simulink model "pasp_16i16c128s"  (Simulink 6.2)
settings: Solver=ode45  StartTime=0.0  StopTime=30000  RelTol=1e-3
undefined symbols (not defined in the file or in its folder): iBOB
libraries: xbsIndex_r3 x1501, casper_library x145, xps_library x90
(part 5 of 12)

== system pasp_16i16c128s/pasp/pfb_fir_real/pol1_in1_first_tap ==
  din : Inport  Port=1  LatchInput=off
  sync : Inport  Port=2  LatchInput=off
  Mult : xbsIndex_r3/Mult  precision=Full  arith_type="Signed  (2's comp)"  n_bits=8  bin_pt=2  quantization=Truncate  overflow=Wrap  latency=mult_latency  explicit_period=off  period=1  en=off  dbl_ovrd=off  show_param=on  mult_type=Parallel  oversample=2  use_embedded=on  pipeline=on  use_rpm=on  placement_style=Rectangular Shape  gen_core=off
      settings: xl_area=[0, 0, 0, 0, 0, 0, 0]
  Reinterpret : xbsIndex_r3/Reinterpret  force_arith_type=on  arith_type="Signed  (2's comp)"  force_bin_pt=on  bin_pt=CoeffBitWidth - 1  force_valid=on
  Reinterpret1 : xbsIndex_r3/Reinterpret  force_arith_type=on  arith_type=Unsigned  force_bin_pt=on  bin_pt=0  force_valid=on
  Reinterpret2 : xbsIndex_r3/Reinterpret  force_arith_type=on  arith_type="Signed  (2's comp)"  force_bin_pt=on  bin_pt=BitWidthIn - 1  force_valid=on
  Slice : xbsIndex_r3/Slice  mode=Lower Bit Location + Width  nbits=CoeffBitWidth  bit1=0  base1=MSB of Input  bit0=0  base0=LSB of Input  boolean_output=off  explicit_period=off  period=1  dbl_ovrd=off
  Slice1 : xbsIndex_r3/Slice  mode=Two Bit Locations  nbits=CoeffBitWidth * (TotalTaps - 1)  bit1=0  base1=MSB of Input  bit0=CoeffBitWidth  base0=LSB of Input  boolean_output=off  explicit_period=off  period=1  dbl_ovrd=off
  delay : Subsystem  BlockChoice=delay_bram
      link override delay_bram: DelayLen=2^(PFBSize-n_inputs)  bram_latency=bram_latency
      link override delay_bram/Constant2: equ=P=C
      settings: AttributesFormatString=%<BlockChoice>  TemplateBlock=casper_library/Delays/delay  MemberBlocks=delay_bram,delay_slr
  pfb_coeff_gen : Subsystem  AncestorBlock=casper_library/PFBs/pfb_coeff_gen  mask(pfb_coeff_gen){PFBSize=5, CoeffBitWidth=8, TotalTaps=2, CoeffDistMem=1, CoeffRound=0, WindowType=hamming, bram_latency=2, n_inputs=2, nput=0, fwidth=1}
      mask prompts: PFBSize "Size of PFB: (2^? pnts)"; CoeffBitWidth "Bitwidth of Coefficients:"; TotalTaps "Total Number of Taps:"; CoeffDistMem "Implement Coeff Gen in Distributed Memory"; CoeffRound "Round-off Coefficients"; WindowType "Windowing Function:"; bram_latency "BRAM Latency"; n_inputs "Number of Simultaneous Inputs: (2^?)"; nput "This is input number:"; fwidth "Bin Width (normal=1)"
      mask init:
      | pfb_coeff_gen_init(gcb, ...
      |     'PFBSize', PFBSize, ...
      |     'CoeffBitWidth', CoeffBitWidth, ...
      |     'CoeffRound', CoeffRound, ...
      |     'TotalTaps', TotalTaps, ...
      |     'CoeffDistMem', CoeffDistMem, ...
      |     'WindowType', WindowType, ...
      |     'bram_latency', bram_latency, ...
      |     'n_inputs', n_inputs, ...
      |     'nput', nput, ...
      |     'fwidth', fwidth);
      settings: AttributesFormatString=PFBSize=5, n_inputs=2, taps=2
  sync_delay : casper_library/Delays/sync_delay  DelayLen=2^(PFBSize-n_inputs)
      link override Constant: equ=P=C
      link override Constant1: equ=P=C
      link override Constant2: equ=P=C
      link override Constant3: equ=P=C
  dout : Outport
  sync_out : Outport  Port=2
  coeff_out : Outport  Port=3
  taps_out : Outport  Port=4
  wires:
  Reinterpret2/1 -> Mult/1
  Reinterpret1/1 -> taps_out/1
  Reinterpret/1 -> Mult/2
  Slice/1 -> Reinterpret/1
  Slice1/1 -> coeff_out/1
  sync_delay/1 -> sync_out/1
  delay/1(Out1) -> dout/1
  pfb_coeff_gen/1(dout) -> delay/1(In1), Reinterpret2/1
  pfb_coeff_gen/2(sync_out) -> sync_delay/1
  pfb_coeff_gen/3(coeff) -> Slice/1, Slice1/1
  Mult/1 -> Reinterpret1/1
  din/1 -> pfb_coeff_gen/1(din)
  sync/1 -> pfb_coeff_gen/2(sync)

== system pasp_16i16c128s/pasp/pfb_fir_real/pol1_in1_last_tap ==
  din : Inport  Port=1  LatchInput=off
  sync : Inport  Port=2  LatchInput=off
  coeff : Inport  Port=3  LatchInput=off
  taps : Inport  Port=4  LatchInput=off
  Concat : xbsIndex_r3/Concat  num_inputs=2  explicit_period=off  period=1  dbl_ovrd=off
  Delay : xbsIndex_r3/Delay  latency=mult_latency  reg_retiming=off  explicit_period=off  period=1  en=off  accept_only_valid=off  init_zero=on  dbl_ovrd=off  show_param=off
      settings: xl_area=[0, 0, 0, 0, 0, 0, 0]
  Mult : xbsIndex_r3/Mult  precision=Full  arith_type="Signed  (2's comp)"  n_bits=8  bin_pt=2  quantization=Truncate  overflow=Wrap  latency=mult_latency  explicit_period=off  period=1  en=off  dbl_ovrd=off  show_param=on  mult_type=Parallel  oversample=2  use_embedded=on  pipeline=on  use_rpm=on  placement_style=Rectangular Shape  gen_core=off
      settings: xl_area=[0, 0, 0, 0, 0, 0, 0]
  Reinterpret : xbsIndex_r3/Reinterpret  force_arith_type=on  arith_type="Signed  (2's comp)"  force_bin_pt=on  bin_pt=CoeffBitWidth - 1  force_valid=on
  Reinterpret1 : xbsIndex_r3/Reinterpret  force_arith_type=on  arith_type="Signed  (2's comp)"  force_bin_pt=on  bin_pt=BitWidthIn - 1  force_valid=on
  Reinterpret2 : xbsIndex_r3/Reinterpret  force_arith_type=on  arith_type=Unsigned  force_bin_pt=on  bin_pt=0  force_valid=on
  pfb_real_add_tree : Subsystem  mask(pfb_real_add_tree){TotalTaps=2, BitWidthIn=8, BitWidthOut=18, CoeffBitWidth=8, add_latency=1, quantization=Truncate}
      mask prompts: TotalTaps "Total Number of Taps:"; BitWidthIn "Input Bitwidth:"; BitWidthOut "Output Bitwidth:"; CoeffBitWidth "Coeff Bitwidth:"; add_latency "Add Latency"; quantization "Quantization Behavior"
      mask init:
      | pfb_real_add_tree_init(gcb, ...
      |     'TotalTaps', TotalTaps, ...
      |     'BitWidthIn', BitWidthIn, ...
      |     'BitWidthOut', BitWidthOut, ...
      |     'CoeffBitWidth', CoeffBitWidth, ...
      |     'add_latency', add_latency, ...
      |     'quantization', quantization);
      settings: AttributesFormatString=taps=2, add_latency=1
  dout : Outport
  sync_out : Outport  Port=2
  wires:
  Delay/1 -> pfb_real_add_tree/2(sync)
  pfb_real_add_tree/2(sync_out) -> sync_out/1
  din/1 -> Reinterpret1/1
  sync/1 -> Delay/1
  taps/1 -> Concat/2
  Concat/1 -> pfb_real_add_tree/1(din)
  coeff/1 -> Reinterpret/1
  Reinterpret/1 -> Mult/2
  Mult/1 -> Reinterpret2/1
  Reinterpret1/1 -> Mult/1
  Reinterpret2/1 -> Concat/1
  pfb_real_add_tree/1(dout) -> dout/1

== system pasp_16i16c128s/pasp/pfb_fir_real/pol1_in2_first_tap ==
  din : Inport  Port=1  LatchInput=off
  sync : Inport  Port=2  LatchInput=off
  Mult : xbsIndex_r3/Mult  precision=Full  arith_type="Signed  (2's comp)"  n_bits=8  bin_pt=2  quantization=Truncate  overflow=Wrap  latency=mult_latency  explicit_period=off  period=1  en=off  dbl_ovrd=off  show_param=on  mult_type=Parallel  oversample=2  use_embedded=on  pipeline=on  use_rpm=on  placement_style=Rectangular Shape  gen_core=off
      settings: xl_area=[0, 0, 0, 0, 0, 0, 0]
  Reinterpret : xbsIndex_r3/Reinterpret  force_arith_type=on  arith_type="Signed  (2's comp)"  force_bin_pt=on  bin_pt=CoeffBitWidth - 1  force_valid=on
  Reinterpret1 : xbsIndex_r3/Reinterpret  force_arith_type=on  arith_type=Unsigned  force_bin_pt=on  bin_pt=0  force_valid=on
  Reinterpret2 : xbsIndex_r3/Reinterpret  force_arith_type=on  arith_type="Signed  (2's comp)"  force_bin_pt=on  bin_pt=BitWidthIn - 1  force_valid=on
  Slice : xbsIndex_r3/Slice  mode=Lower Bit Location + Width  nbits=CoeffBitWidth  bit1=0  base1=MSB of Input  bit0=0  base0=LSB of Input  boolean_output=off  explicit_period=off  period=1  dbl_ovrd=off
  Slice1 : xbsIndex_r3/Slice  mode=Two Bit Locations  nbits=CoeffBitWidth * (TotalTaps - 1)  bit1=0  base1=MSB of Input  bit0=CoeffBitWidth  base0=LSB of Input  boolean_output=off  explicit_period=off  period=1  dbl_ovrd=off
  delay : Subsystem  BlockChoice=delay_bram
      link override delay_bram: DelayLen=2^(PFBSize-n_inputs)  bram_latency=bram_latency
      link override delay_bram/Constant2: equ=P=C
      settings: AttributesFormatString=%<BlockChoice>  TemplateBlock=casper_library/Delays/delay  MemberBlocks=delay_bram,delay_slr
  pfb_coeff_gen : Subsystem  AncestorBlock=casper_library/PFBs/pfb_coeff_gen  mask(pfb_coeff_gen){PFBSize=5, CoeffBitWidth=8, TotalTaps=2, CoeffDistMem=1, CoeffRound=0, WindowType=hamming, bram_latency=2, n_inputs=2, nput=1, fwidth=1}
      mask prompts: PFBSize "Size of PFB: (2^? pnts)"; CoeffBitWidth "Bitwidth of Coefficients:"; TotalTaps "Total Number of Taps:"; CoeffDistMem "Implement Coeff Gen in Distributed Memory"; CoeffRound "Round-off Coefficients"; WindowType "Windowing Function:"; bram_latency "BRAM Latency"; n_inputs "Number of Simultaneous Inputs: (2^?)"; nput "This is input number:"; fwidth "Bin Width (normal=1)"
      mask init: same as pasp_16i16c128s/pasp/pfb_fir_real/pol1_in1_first_tap/pfb_coeff_gen
      settings: AttributesFormatString=PFBSize=5, n_inputs=2, taps=2
  sync_delay : casper_library/Delays/sync_delay  DelayLen=2^(PFBSize-n_inputs)
      link override Constant: equ=P=C
      link override Constant1: equ=P=C
      link override Constant2: equ=P=C
      link override Constant3: equ=P=C
  dout : Outport
  sync_out : Outport  Port=2
  coeff_out : Outport  Port=3
  taps_out : Outport  Port=4
  wires:
  Reinterpret2/1 -> Mult/1
  Reinterpret1/1 -> taps_out/1
  Reinterpret/1 -> Mult/2
  Slice/1 -> Reinterpret/1
  Slice1/1 -> coeff_out/1
  sync_delay/1 -> sync_out/1
  delay/1(Out1) -> dout/1
  pfb_coeff_gen/1(dout) -> delay/1(In1), Reinterpret2/1
  pfb_coeff_gen/2(sync_out) -> sync_delay/1
  pfb_coeff_gen/3(coeff) -> Slice/1, Slice1/1
  Mult/1 -> Reinterpret1/1
  din/1 -> pfb_coeff_gen/1(din)
  sync/1 -> pfb_coeff_gen/2(sync)

== system pasp_16i16c128s/pasp/pfb_fir_real/pol1_in2_last_tap ==
  din : Inport  Port=1  LatchInput=off
  sync : Inport  Port=2  LatchInput=off
  coeff : Inport  Port=3  LatchInput=off
  taps : Inport  Port=4  LatchInput=off
  Concat : xbsIndex_r3/Concat  num_inputs=2  explicit_period=off  period=1  dbl_ovrd=off
  Delay : xbsIndex_r3/Delay  latency=mult_latency  reg_retiming=off  explicit_period=off  period=1  en=off  accept_only_valid=off  init_zero=on  dbl_ovrd=off  show_param=off
      settings: xl_area=[0, 0, 0, 0, 0, 0, 0]
  Mult : xbsIndex_r3/Mult  precision=Full  arith_type="Signed  (2's comp)"  n_bits=8  bin_pt=2  quantization=Truncate  overflow=Wrap  latency=mult_latency  explicit_period=off  period=1  en=off  dbl_ovrd=off  show_param=on  mult_type=Parallel  oversample=2  use_embedded=on  pipeline=on  use_rpm=on  placement_style=Rectangular Shape  gen_core=off
      settings: xl_area=[0, 0, 0, 0, 0, 0, 0]
  Reinterpret : xbsIndex_r3/Reinterpret  force_arith_type=on  arith_type="Signed  (2's comp)"  force_bin_pt=on  bin_pt=CoeffBitWidth - 1  force_valid=on
  Reinterpret1 : xbsIndex_r3/Reinterpret  force_arith_type=on  arith_type="Signed  (2's comp)"  force_bin_pt=on  bin_pt=BitWidthIn - 1  force_valid=on
  Reinterpret2 : xbsIndex_r3/Reinterpret  force_arith_type=on  arith_type=Unsigned  force_bin_pt=on  bin_pt=0  force_valid=on
  pfb_real_add_tree : Subsystem  mask(pfb_real_add_tree){TotalTaps=2, BitWidthIn=8, BitWidthOut=18, CoeffBitWidth=8, add_latency=1, quantization=Truncate}
      mask prompts: TotalTaps "Total Number of Taps:"; BitWidthIn "Input Bitwidth:"; BitWidthOut "Output Bitwidth:"; CoeffBitWidth "Coeff Bitwidth:"; add_latency "Add Latency"; quantization "Quantization Behavior"
      mask init: same as pasp_16i16c128s/pasp/pfb_fir_real/pol1_in1_last_tap/pfb_real_add_tree
      settings: AttributesFormatString=taps=2, add_latency=1
  dout : Outport
  sync_out : Outport  Port=2
  wires:
  Delay/1 -> pfb_real_add_tree/2(sync)
  pfb_real_add_tree/2(sync_out) -> sync_out/1
  din/1 -> Reinterpret1/1
  sync/1 -> Delay/1
  taps/1 -> Concat/2
  Concat/1 -> pfb_real_add_tree/1(din)
  coeff/1 -> Reinterpret/1
  Reinterpret/1 -> Mult/2
  Mult/1 -> Reinterpret2/1
  Reinterpret1/1 -> Mult/1
  Reinterpret2/1 -> Concat/1
  pfb_real_add_tree/1(dout) -> dout/1

== system pasp_16i16c128s/pasp/pfb_fir_real/pol1_in3_first_tap ==
  din : Inport  Port=1  LatchInput=off
  sync : Inport  Port=2  LatchInput=off
  Mult : xbsIndex_r3/Mult  precision=Full  arith_type="Signed  (2's comp)"  n_bits=8  bin_pt=2  quantization=Truncate  overflow=Wrap  latency=mult_latency  explicit_period=off  period=1  en=off  dbl_ovrd=off  show_param=on  mult_type=Parallel  oversample=2  use_embedded=on  pipeline=on  use_rpm=on  placement_style=Rectangular Shape  gen_core=off
      settings: xl_area=[0, 0, 0, 0, 0, 0, 0]
  Reinterpret : xbsIndex_r3/Reinterpret  force_arith_type=on  arith_type="Signed  (2's comp)"  force_bin_pt=on  bin_pt=CoeffBitWidth - 1  force_valid=on
  Reinterpret1 : xbsIndex_r3/Reinterpret  force_arith_type=on  arith_type=Unsigned  force_bin_pt=on  bin_pt=0  force_valid=on
  Reinterpret2 : xbsIndex_r3/Reinterpret  force_arith_type=on  arith_type="Signed  (2's comp)"  force_bin_pt=on  bin_pt=BitWidthIn - 1  force_valid=on
  Slice : xbsIndex_r3/Slice  mode=Lower Bit Location + Width  nbits=CoeffBitWidth  bit1=0  base1=MSB of Input  bit0=0  base0=LSB of Input  boolean_output=off  explicit_period=off  period=1  dbl_ovrd=off
  Slice1 : xbsIndex_r3/Slice  mode=Two Bit Locations  nbits=CoeffBitWidth * (TotalTaps - 1)  bit1=0  base1=MSB of Input  bit0=CoeffBitWidth  base0=LSB of Input  boolean_output=off  explicit_period=off  period=1  dbl_ovrd=off
  delay : Subsystem  BlockChoice=delay_bram
      link override delay_bram: DelayLen=2^(PFBSize-n_inputs)  bram_latency=bram_latency
      link override delay_bram/Constant2: equ=P=C
      settings: AttributesFormatString=%<BlockChoice>  TemplateBlock=casper_library/Delays/delay  MemberBlocks=delay_bram,delay_slr
  pfb_coeff_gen : Subsystem  AncestorBlock=casper_library/PFBs/pfb_coeff_gen  mask(pfb_coeff_gen){PFBSize=5, CoeffBitWidth=8, TotalTaps=2, CoeffDistMem=1, CoeffRound=0, WindowType=hamming, bram_latency=2, n_inputs=2, nput=2, fwidth=1}
      mask prompts: PFBSize "Size of PFB: (2^? pnts)"; CoeffBitWidth "Bitwidth of Coefficients:"; TotalTaps "Total Number of Taps:"; CoeffDistMem "Implement Coeff Gen in Distributed Memory"; CoeffRound "Round-off Coefficients"; WindowType "Windowing Function:"; bram_latency "BRAM Latency"; n_inputs "Number of Simultaneous Inputs: (2^?)"; nput "This is input number:"; fwidth "Bin Width (normal=1)"
      mask init: same as pasp_16i16c128s/pasp/pfb_fir_real/pol1_in1_first_tap/pfb_coeff_gen
      settings: AttributesFormatString=PFBSize=5, n_inputs=2, taps=2
  sync_delay : casper_library/Delays/sync_delay  DelayLen=2^(PFBSize-n_inputs)
      link override Constant: equ=P=C
      link override Constant1: equ=P=C
      link override Constant2: equ=P=C
      link override Constant3: equ=P=C
  dout : Outport
  sync_out : Outport  Port=2
  coeff_out : Outport  Port=3
  taps_out : Outport  Port=4
  wires:
  Reinterpret2/1 -> Mult/1
  Reinterpret1/1 -> taps_out/1
  Reinterpret/1 -> Mult/2
  Slice/1 -> Reinterpret/1
  Slice1/1 -> coeff_out/1
  sync_delay/1 -> sync_out/1
  delay/1(Out1) -> dout/1
  pfb_coeff_gen/1(dout) -> delay/1(In1), Reinterpret2/1
  pfb_coeff_gen/2(sync_out) -> sync_delay/1
  pfb_coeff_gen/3(coeff) -> Slice/1, Slice1/1
  Mult/1 -> Reinterpret1/1
  din/1 -> pfb_coeff_gen/1(din)
  sync/1 -> pfb_coeff_gen/2(sync)

== system pasp_16i16c128s/pasp/pfb_fir_real/pol1_in3_last_tap ==
  din : Inport  Port=1  LatchInput=off
  sync : Inport  Port=2  LatchInput=off
  coeff : Inport  Port=3  LatchInput=off
  taps : Inport  Port=4  LatchInput=off
  Concat : xbsIndex_r3/Concat  num_inputs=2  explicit_period=off  period=1  dbl_ovrd=off
  Delay : xbsIndex_r3/Delay  latency=mult_latency  reg_retiming=off  explicit_period=off  period=1  en=off  accept_only_valid=off  init_zero=on  dbl_ovrd=off  show_param=off
      settings: xl_area=[0, 0, 0, 0, 0, 0, 0]
  Mult : xbsIndex_r3/Mult  precision=Full  arith_type="Signed  (2's comp)"  n_bits=8  bin_pt=2  quantization=Truncate  overflow=Wrap  latency=mult_latency  explicit_period=off  period=1  en=off  dbl_ovrd=off  show_param=on  mult_type=Parallel  oversample=2  use_embedded=on  pipeline=on  use_rpm=on  placement_style=Rectangular Shape  gen_core=off
      settings: xl_area=[0, 0, 0, 0, 0, 0, 0]
  Reinterpret : xbsIndex_r3/Reinterpret  force_arith_type=on  arith_type="Signed  (2's comp)"  force_bin_pt=on  bin_pt=CoeffBitWidth - 1  force_valid=on
  Reinterpret1 : xbsIndex_r3/Reinterpret  force_arith_type=on  arith_type="Signed  (2's comp)"  force_bin_pt=on  bin_pt=BitWidthIn - 1  force_valid=on
  Reinterpret2 : xbsIndex_r3/Reinterpret  force_arith_type=on  arith_type=Unsigned  force_bin_pt=on  bin_pt=0  force_valid=on
  pfb_real_add_tree : Subsystem  mask(pfb_real_add_tree){TotalTaps=2, BitWidthIn=8, BitWidthOut=18, CoeffBitWidth=8, add_latency=1, quantization=Truncate}
      mask prompts: TotalTaps "Total Number of Taps:"; BitWidthIn "Input Bitwidth:"; BitWidthOut "Output Bitwidth:"; CoeffBitWidth "Coeff Bitwidth:"; add_latency "Add Latency"; quantization "Quantization Behavior"
      mask init: same as pasp_16i16c128s/pasp/pfb_fir_real/pol1_in1_last_tap/pfb_real_add_tree
      settings: AttributesFormatString=taps=2, add_latency=1
  dout : Outport
  sync_out : Outport  Port=2
  wires:
  Delay/1 -> pfb_real_add_tree/2(sync)
  pfb_real_add_tree/2(sync_out) -> sync_out/1
  din/1 -> Reinterpret1/1
  sync/1 -> Delay/1
  taps/1 -> Concat/2
  Concat/1 -> pfb_real_add_tree/1(din)
  coeff/1 -> Reinterpret/1
  Reinterpret/1 -> Mult/2
  Mult/1 -> Reinterpret2/1
  Reinterpret1/1 -> Mult/1
  Reinterpret2/1 -> Concat/1
  pfb_real_add_tree/1(dout) -> dout/1

== system pasp_16i16c128s/pasp/pfb_fir_real/pol1_in4_first_tap ==
  din : Inport  Port=1  LatchInput=off
  sync : Inport  Port=2  LatchInput=off
  Mult : xbsIndex_r3/Mult  precision=Full  arith_type="Signed  (2's comp)"  n_bits=8  bin_pt=2  quantization=Truncate  overflow=Wrap  latency=mult_latency  explicit_period=off  period=1  en=off  dbl_ovrd=off  show_param=on  mult_type=Parallel  oversample=2  use_embedded=on  pipeline=on  use_rpm=on  placement_style=Rectangular Shape  gen_core=off
      settings: xl_area=[0, 0, 0, 0, 0, 0, 0]
  Reinterpret : xbsIndex_r3/Reinterpret  force_arith_type=on  arith_type="Signed  (2's comp)"  force_bin_pt=on  bin_pt=CoeffBitWidth - 1  force_valid=on
  Reinterpret1 : xbsIndex_r3/Reinterpret  force_arith_type=on  arith_type=Unsigned  force_bin_pt=on  bin_pt=0  force_valid=on
  Reinterpret2 : xbsIndex_r3/Reinterpret  force_arith_type=on  arith_type="Signed  (2's comp)"  force_bin_pt=on  bin_pt=BitWidthIn - 1  force_valid=on
  Slice : xbsIndex_r3/Slice  mode=Lower Bit Location + Width  nbits=CoeffBitWidth  bit1=0  base1=MSB of Input  bit0=0  base0=LSB of Input  boolean_output=off  explicit_period=off  period=1  dbl_ovrd=off
  Slice1 : xbsIndex_r3/Slice  mode=Two Bit Locations  nbits=CoeffBitWidth * (TotalTaps - 1)  bit1=0  base1=MSB of Input  bit0=CoeffBitWidth  base0=LSB of Input  boolean_output=off  explicit_period=off  period=1  dbl_ovrd=off
  delay : Subsystem  BlockChoice=delay_bram
      link override delay_bram: DelayLen=2^(PFBSize-n_inputs)  bram_latency=bram_latency
      link override delay_bram/Constant2: equ=P=C
      settings: AttributesFormatString=%<BlockChoice>  TemplateBlock=casper_library/Delays/delay  MemberBlocks=delay_bram,delay_slr
  pfb_coeff_gen : Subsystem  AncestorBlock=casper_library/PFBs/pfb_coeff_gen  mask(pfb_coeff_gen){PFBSize=5, CoeffBitWidth=8, TotalTaps=2, CoeffDistMem=1, CoeffRound=0, WindowType=hamming, bram_latency=2, n_inputs=2, nput=3, fwidth=1}
      mask prompts: PFBSize "Size of PFB: (2^? pnts)"; CoeffBitWidth "Bitwidth of Coefficients:"; TotalTaps "Total Number of Taps:"; CoeffDistMem "Implement Coeff Gen in Distributed Memory"; CoeffRound "Round-off Coefficients"; WindowType "Windowing Function:"; bram_latency "BRAM Latency"; n_inputs "Number of Simultaneous Inputs: (2^?)"; nput "This is input number:"; fwidth "Bin Width (normal=1)"
      mask init: same as pasp_16i16c128s/pasp/pfb_fir_real/pol1_in1_first_tap/pfb_coeff_gen
      settings: AttributesFormatString=PFBSize=5, n_inputs=2, taps=2
  sync_delay : casper_library/Delays/sync_delay  DelayLen=2^(PFBSize-n_inputs)
      link override Constant: equ=P=C
      link override Constant1: equ=P=C
      link override Constant2: equ=P=C
      link override Constant3: equ=P=C
  dout : Outport
  sync_out : Outport  Port=2
  coeff_out : Outport  Port=3
  taps_out : Outport  Port=4
  wires:
  Reinterpret2/1 -> Mult/1
  Reinterpret1/1 -> taps_out/1
  Reinterpret/1 -> Mult/2
  Slice/1 -> Reinterpret/1
  Slice1/1 -> coeff_out/1
  sync_delay/1 -> sync_out/1
  delay/1(Out1) -> dout/1
  pfb_coeff_gen/1(dout) -> delay/1(In1), Reinterpret2/1
  pfb_coeff_gen/2(sync_out) -> sync_delay/1
  pfb_coeff_gen/3(coeff) -> Slice/1, Slice1/1
  Mult/1 -> Reinterpret1/1
  din/1 -> pfb_coeff_gen/1(din)
  sync/1 -> pfb_coeff_gen/2(sync)

== system pasp_16i16c128s/pasp/pfb_fir_real/pol1_in4_last_tap ==
  din : Inport  Port=1  LatchInput=off
  sync : Inport  Port=2  LatchInput=off
  coeff : Inport  Port=3  LatchInput=off
  taps : Inport  Port=4  LatchInput=off
  Concat : xbsIndex_r3/Concat  num_inputs=2  explicit_period=off  period=1  dbl_ovrd=off
  Delay : xbsIndex_r3/Delay  latency=mult_latency  reg_retiming=off  explicit_period=off  period=1  en=off  accept_only_valid=off  init_zero=on  dbl_ovrd=off  show_param=off
      settings: xl_area=[0, 0, 0, 0, 0, 0, 0]
  Mult : xbsIndex_r3/Mult  precision=Full  arith_type="Signed  (2's comp)"  n_bits=8  bin_pt=2  quantization=Truncate  overflow=Wrap  latency=mult_latency  explicit_period=off  period=1  en=off  dbl_ovrd=off  show_param=on  mult_type=Parallel  oversample=2  use_embedded=on  pipeline=on  use_rpm=on  placement_style=Rectangular Shape  gen_core=off
      settings: xl_area=[0, 0, 0, 0, 0, 0, 0]
  Reinterpret : xbsIndex_r3/Reinterpret  force_arith_type=on  arith_type="Signed  (2's comp)"  force_bin_pt=on  bin_pt=CoeffBitWidth - 1  force_valid=on
  Reinterpret1 : xbsIndex_r3/Reinterpret  force_arith_type=on  arith_type="Signed  (2's comp)"  force_bin_pt=on  bin_pt=BitWidthIn - 1  force_valid=on
  Reinterpret2 : xbsIndex_r3/Reinterpret  force_arith_type=on  arith_type=Unsigned  force_bin_pt=on  bin_pt=0  force_valid=on
  pfb_real_add_tree : Subsystem  mask(pfb_real_add_tree){TotalTaps=2, BitWidthIn=8, BitWidthOut=18, CoeffBitWidth=8, add_latency=1, quantization=Truncate}
      mask prompts: TotalTaps "Total Number of Taps:"; BitWidthIn "Input Bitwidth:"; BitWidthOut "Output Bitwidth:"; CoeffBitWidth "Coeff Bitwidth:"; add_latency "Add Latency"; quantization "Quantization Behavior"
      mask init: same as pasp_16i16c128s/pasp/pfb_fir_real/pol1_in1_last_tap/pfb_real_add_tree
      settings: AttributesFormatString=taps=2, add_latency=1
  dout : Outport
  sync_out : Outport  Port=2
  wires:
  Delay/1 -> pfb_real_add_tree/2(sync)
  pfb_real_add_tree/2(sync_out) -> sync_out/1
  din/1 -> Reinterpret1/1
  sync/1 -> Delay/1
  taps/1 -> Concat/2
  Concat/1 -> pfb_real_add_tree/1(din)
  coeff/1 -> Reinterpret/1
  Reinterpret/1 -> Mult/2
  Mult/1 -> Reinterpret2/1
  Reinterpret1/1 -> Mult/1
  Reinterpret2/1 -> Concat/1
  pfb_real_add_tree/1(dout) -> dout/1

== system pasp_16i16c128s/pasp/pfb_fir_real1/pol1_in1_first_tap ==
  din : Inport  Port=1  LatchInput=off
  sync : Inport  Port=2  LatchInput=off
  Mult : xbsIndex_r3/Mult  precision=Full  arith_type="Signed  (2's comp)"  n_bits=8  bin_pt=2  quantization=Truncate  overflow=Wrap  latency=mult_latency  explicit_period=off  period=1  en=off  dbl_ovrd=off  show_param=on  mult_type=Parallel  oversample=2  use_embedded=on  pipeline=on  use_rpm=on  placement_style=Rectangular Shape  gen_core=off
      settings: xl_area=[0, 0, 0, 0, 0, 0, 0]
  Reinterpret : xbsIndex_r3/Reinterpret  force_arith_type=on  arith_type="Signed  (2's comp)"  force_bin_pt=on  bin_pt=CoeffBitWidth - 1  force_valid=on
  Reinterpret1 : xbsIndex_r3/Reinterpret  force_arith_type=on  arith_type=Unsigned  force_bin_pt=on  bin_pt=0  force_valid=on
  Reinterpret2 : xbsIndex_r3/Reinterpret  force_arith_type=on  arith_type="Signed  (2's comp)"  force_bin_pt=on  bin_pt=BitWidthIn - 1  force_valid=on
  Slice : xbsIndex_r3/Slice  mode=Lower Bit Location + Width  nbits=CoeffBitWidth  bit1=0  base1=MSB of Input  bit0=0  base0=LSB of Input  boolean_output=off  explicit_period=off  period=1  dbl_ovrd=off
  Slice1 : xbsIndex_r3/Slice  mode=Two Bit Locations  nbits=CoeffBitWidth * (TotalTaps - 1)  bit1=0  base1=MSB of Input  bit0=CoeffBitWidth  base0=LSB of Input  boolean_output=off  explicit_period=off  period=1  dbl_ovrd=off
  delay : Subsystem  BlockChoice=delay_bram
      link override delay_bram: DelayLen=2^(PFBSize-n_inputs)  bram_latency=bram_latency
      link override delay_bram/Constant2: equ=P=C
      settings: AttributesFormatString=%<BlockChoice>  TemplateBlock=casper_library/Delays/delay  MemberBlocks=delay_bram,delay_slr
  pfb_coeff_gen : Subsystem  AncestorBlock=casper_library/PFBs/pfb_coeff_gen  mask(pfb_coeff_gen){PFBSize=5, CoeffBitWidth=8, TotalTaps=2, CoeffDistMem=1, CoeffRound=0, WindowType=hamming, bram_latency=2, n_inputs=2, nput=0, fwidth=1}
      mask prompts: PFBSize "Size of PFB: (2^? pnts)"; CoeffBitWidth "Bitwidth of Coefficients:"; TotalTaps "Total Number of Taps:"; CoeffDistMem "Implement Coeff Gen in Distributed Memory"; CoeffRound "Round-off Coefficients"; WindowType "Windowing Function:"; bram_latency "BRAM Latency"; n_inputs "Number of Simultaneous Inputs: (2^?)"; nput "This is input number:"; fwidth "Bin Width (normal=1)"
      mask init: same as pasp_16i16c128s/pasp/pfb_fir_real/pol1_in1_first_tap/pfb_coeff_gen
      settings: AttributesFormatString=PFBSize=5, n_inputs=2, taps=2
  sync_delay : casper_library/Delays/sync_delay  DelayLen=2^(PFBSize-n_inputs)
      link override Constant: equ=P=C
      link override Constant1: equ=P=C
      link override Constant2: equ=P=C
      link override Constant3: equ=P=C
  dout : Outport
  sync_out : Outport  Port=2
  coeff_out : Outport  Port=3
  taps_out : Outport  Port=4
  wires:
  Reinterpret2/1 -> Mult/1
  Reinterpret1/1 -> taps_out/1
  Reinterpret/1 -> Mult/2
  Slice/1 -> Reinterpret/1
  Slice1/1 -> coeff_out/1
  sync_delay/1 -> sync_out/1
  delay/1(Out1) -> dout/1
  pfb_coeff_gen/1(dout) -> delay/1(In1), Reinterpret2/1
  pfb_coeff_gen/2(sync_out) -> sync_delay/1
  pfb_coeff_gen/3(coeff) -> Slice/1, Slice1/1
  Mult/1 -> Reinterpret1/1
  din/1 -> pfb_coeff_gen/1(din)
  sync/1 -> pfb_coeff_gen/2(sync)

== system pasp_16i16c128s/pasp/pfb_fir_real1/pol1_in1_last_tap ==
  din : Inport  Port=1  LatchInput=off
  sync : Inport  Port=2  LatchInput=off
  coeff : Inport  Port=3  LatchInput=off
  taps : Inport  Port=4  LatchInput=off
  Concat : xbsIndex_r3/Concat  num_inputs=2  explicit_period=off  period=1  dbl_ovrd=off
  Delay : xbsIndex_r3/Delay  latency=mult_latency  reg_retiming=off  explicit_period=off  period=1  en=off  accept_only_valid=off  init_zero=on  dbl_ovrd=off  show_param=off
      settings: xl_area=[0, 0, 0, 0, 0, 0, 0]
  Mult : xbsIndex_r3/Mult  precision=Full  arith_type="Signed  (2's comp)"  n_bits=8  bin_pt=2  quantization=Truncate  overflow=Wrap  latency=mult_latency  explicit_period=off  period=1  en=off  dbl_ovrd=off  show_param=on  mult_type=Parallel  oversample=2  use_embedded=on  pipeline=on  use_rpm=on  placement_style=Rectangular Shape  gen_core=off
      settings: xl_area=[0, 0, 0, 0, 0, 0, 0]
  Reinterpret : xbsIndex_r3/Reinterpret  force_arith_type=on  arith_type="Signed  (2's comp)"  force_bin_pt=on  bin_pt=CoeffBitWidth - 1  force_valid=on
  Reinterpret1 : xbsIndex_r3/Reinterpret  force_arith_type=on  arith_type="Signed  (2's comp)"  force_bin_pt=on  bin_pt=BitWidthIn - 1  force_valid=on
  Reinterpret2 : xbsIndex_r3/Reinterpret  force_arith_type=on  arith_type=Unsigned  force_bin_pt=on  bin_pt=0  force_valid=on
  pfb_real_add_tree : Subsystem  mask(pfb_real_add_tree){TotalTaps=2, BitWidthIn=8, BitWidthOut=18, CoeffBitWidth=8, add_latency=1, quantization=Truncate}
      mask prompts: TotalTaps "Total Number of Taps:"; BitWidthIn "Input Bitwidth:"; BitWidthOut "Output Bitwidth:"; CoeffBitWidth "Coeff Bitwidth:"; add_latency "Add Latency"; quantization "Quantization Behavior"
      mask init: same as pasp_16i16c128s/pasp/pfb_fir_real/pol1_in1_last_tap/pfb_real_add_tree
      settings: AttributesFormatString=taps=2, add_latency=1
  dout : Outport
  sync_out : Outport  Port=2
  wires:
  Delay/1 -> pfb_real_add_tree/2(sync)
  pfb_real_add_tree/2(sync_out) -> sync_out/1
  din/1 -> Reinterpret1/1
  sync/1 -> Delay/1
  taps/1 -> Concat/2
  Concat/1 -> pfb_real_add_tree/1(din)
  coeff/1 -> Reinterpret/1
  Reinterpret/1 -> Mult/2
  Mult/1 -> Reinterpret2/1
  Reinterpret1/1 -> Mult/1
  Reinterpret2/1 -> Concat/1
  pfb_real_add_tree/1(dout) -> dout/1

== system pasp_16i16c128s/pasp/pfb_fir_real1/pol1_in2_first_tap ==
  din : Inport  Port=1  LatchInput=off
  sync : Inport  Port=2  LatchInput=off
  Mult : xbsIndex_r3/Mult  precision=Full  arith_type="Signed  (2's comp)"  n_bits=8  bin_pt=2  quantization=Truncate  overflow=Wrap  latency=mult_latency  explicit_period=off  period=1  en=off  dbl_ovrd=off  show_param=on  mult_type=Parallel  oversample=2  use_embedded=on  pipeline=on  use_rpm=on  placement_style=Rectangular Shape  gen_core=off
      settings: xl_area=[0, 0, 0, 0, 0, 0, 0]
  Reinterpret : xbsIndex_r3/Reinterpret  force_arith_type=on  arith_type="Signed  (2's comp)"  force_bin_pt=on  bin_pt=CoeffBitWidth - 1  force_valid=on
  Reinterpret1 : xbsIndex_r3/Reinterpret  force_arith_type=on  arith_type=Unsigned  force_bin_pt=on  bin_pt=0  force_valid=on
  Reinterpret2 : xbsIndex_r3/Reinterpret  force_arith_type=on  arith_type="Signed  (2's comp)"  force_bin_pt=on  bin_pt=BitWidthIn - 1  force_valid=on
  Slice : xbsIndex_r3/Slice  mode=Lower Bit Location + Width  nbits=CoeffBitWidth  bit1=0  base1=MSB of Input  bit0=0  base0=LSB of Input  boolean_output=off  explicit_period=off  period=1  dbl_ovrd=off
  Slice1 : xbsIndex_r3/Slice  mode=Two Bit Locations  nbits=CoeffBitWidth * (TotalTaps - 1)  bit1=0  base1=MSB of Input  bit0=CoeffBitWidth  base0=LSB of Input  boolean_output=off  explicit_period=off  period=1  dbl_ovrd=off
  delay : Subsystem  BlockChoice=delay_bram
      link override delay_bram: DelayLen=2^(PFBSize-n_inputs)  bram_latency=bram_latency
      link override delay_bram/Constant2: equ=P=C
      settings: AttributesFormatString=%<BlockChoice>  TemplateBlock=casper_library/Delays/delay  MemberBlocks=delay_bram,delay_slr
  pfb_coeff_gen : Subsystem  AncestorBlock=casper_library/PFBs/pfb_coeff_gen  mask(pfb_coeff_gen){PFBSize=5, CoeffBitWidth=8, TotalTaps=2, CoeffDistMem=1, CoeffRound=0, WindowType=hamming, bram_latency=2, n_inputs=2, nput=1, fwidth=1}
      mask prompts: PFBSize "Size of PFB: (2^? pnts)"; CoeffBitWidth "Bitwidth of Coefficients:"; TotalTaps "Total Number of Taps:"; CoeffDistMem "Implement Coeff Gen in Distributed Memory"; CoeffRound "Round-off Coefficients"; WindowType "Windowing Function:"; bram_latency "BRAM Latency"; n_inputs "Number of Simultaneous Inputs: (2^?)"; nput "This is input number:"; fwidth "Bin Width (normal=1)"
      mask init: same as pasp_16i16c128s/pasp/pfb_fir_real/pol1_in1_first_tap/pfb_coeff_gen
      settings: AttributesFormatString=PFBSize=5, n_inputs=2, taps=2
  sync_delay : casper_library/Delays/sync_delay  DelayLen=2^(PFBSize-n_inputs)
      link override Constant: equ=P=C
      link override Constant1: equ=P=C
      link override Constant2: equ=P=C
      link override Constant3: equ=P=C
  dout : Outport
  sync_out : Outport  Port=2
  coeff_out : Outport  Port=3
  taps_out : Outport  Port=4
  wires:
  Reinterpret2/1 -> Mult/1
  Reinterpret1/1 -> taps_out/1
  Reinterpret/1 -> Mult/2
  Slice/1 -> Reinterpret/1
  Slice1/1 -> coeff_out/1
  sync_delay/1 -> sync_out/1
  delay/1(Out1) -> dout/1
  pfb_coeff_gen/1(dout) -> delay/1(In1), Reinterpret2/1
  pfb_coeff_gen/2(sync_out) -> sync_delay/1
  pfb_coeff_gen/3(coeff) -> Slice/1, Slice1/1
  Mult/1 -> Reinterpret1/1
  din/1 -> pfb_coeff_gen/1(din)
  sync/1 -> pfb_coeff_gen/2(sync)

== system pasp_16i16c128s/pasp/pfb_fir_real1/pol1_in2_last_tap ==
  din : Inport  Port=1  LatchInput=off
  sync : Inport  Port=2  LatchInput=off
  coeff : Inport  Port=3  LatchInput=off
  taps : Inport  Port=4  LatchInput=off
  Concat : xbsIndex_r3/Concat  num_inputs=2  explicit_period=off  period=1  dbl_ovrd=off
  Delay : xbsIndex_r3/Delay  latency=mult_latency  reg_retiming=off  explicit_period=off  period=1  en=off  accept_only_valid=off  init_zero=on  dbl_ovrd=off  show_param=off
      settings: xl_area=[0, 0, 0, 0, 0, 0, 0]
  Mult : xbsIndex_r3/Mult  precision=Full  arith_type="Signed  (2's comp)"  n_bits=8  bin_pt=2  quantization=Truncate  overflow=Wrap  latency=mult_latency  explicit_period=off  period=1  en=off  dbl_ovrd=off  show_param=on  mult_type=Parallel  oversample=2  use_embedded=on  pipeline=on  use_rpm=on  placement_style=Rectangular Shape  gen_core=off
      settings: xl_area=[0, 0, 0, 0, 0, 0, 0]
  Reinterpret : xbsIndex_r3/Reinterpret  force_arith_type=on  arith_type="Signed  (2's comp)"  force_bin_pt=on  bin_pt=CoeffBitWidth - 1  force_valid=on
  Reinterpret1 : xbsIndex_r3/Reinterpret  force_arith_type=on  arith_type="Signed  (2's comp)"  force_bin_pt=on  bin_pt=BitWidthIn - 1  force_valid=on
  Reinterpret2 : xbsIndex_r3/Reinterpret  force_arith_type=on  arith_type=Unsigned  force_bin_pt=on  bin_pt=0  force_valid=on
  pfb_real_add_tree : Subsystem  mask(pfb_real_add_tree){TotalTaps=2, BitWidthIn=8, BitWidthOut=18, CoeffBitWidth=8, add_latency=1, quantization=Truncate}
      mask prompts: TotalTaps "Total Number of Taps:"; BitWidthIn "Input Bitwidth:"; BitWidthOut "Output Bitwidth:"; CoeffBitWidth "Coeff Bitwidth:"; add_latency "Add Latency"; quantization "Quantization Behavior"
      mask init: same as pasp_16i16c128s/pasp/pfb_fir_real/pol1_in1_last_tap/pfb_real_add_tree
      settings: AttributesFormatString=taps=2, add_latency=1
  dout : Outport
  sync_out : Outport  Port=2
  wires:
  Delay/1 -> pfb_real_add_tree/2(sync)
  pfb_real_add_tree/2(sync_out) -> sync_out/1
  din/1 -> Reinterpret1/1
  sync/1 -> Delay/1
  taps/1 -> Concat/2
  Concat/1 -> pfb_real_add_tree/1(din)
  coeff/1 -> Reinterpret/1
  Reinterpret/1 -> Mult/2
  Mult/1 -> Reinterpret2/1
  Reinterpret1/1 -> Mult/1
  Reinterpret2/1 -> Concat/1
  pfb_real_add_tree/1(dout) -> dout/1

== system pasp_16i16c128s/pasp/pfb_fir_real1/pol1_in3_first_tap ==
  din : Inport  Port=1  LatchInput=off
  sync : Inport  Port=2  LatchInput=off
  Mult : xbsIndex_r3/Mult  precision=Full  arith_type="Signed  (2's comp)"  n_bits=8  bin_pt=2  quantization=Truncate  overflow=Wrap  latency=mult_latency  explicit_period=off  period=1  en=off  dbl_ovrd=off  show_param=on  mult_type=Parallel  oversample=2  use_embedded=on  pipeline=on  use_rpm=on  placement_style=Rectangular Shape  gen_core=off
      settings: xl_area=[0, 0, 0, 0, 0, 0, 0]
  Reinterpret : xbsIndex_r3/Reinterpret  force_arith_type=on  arith_type="Signed  (2's comp)"  force_bin_pt=on  bin_pt=CoeffBitWidth - 1  force_valid=on
  Reinterpret1 : xbsIndex_r3/Reinterpret  force_arith_type=on  arith_type=Unsigned  force_bin_pt=on  bin_pt=0  force_valid=on
  Reinterpret2 : xbsIndex_r3/Reinterpret  force_arith_type=on  arith_type="Signed  (2's comp)"  force_bin_pt=on  bin_pt=BitWidthIn - 1  force_valid=on
  Slice : xbsIndex_r3/Slice  mode=Lower Bit Location + Width  nbits=CoeffBitWidth  bit1=0  base1=MSB of Input  bit0=0  base0=LSB of Input  boolean_output=off  explicit_period=off  period=1  dbl_ovrd=off
  Slice1 : xbsIndex_r3/Slice  mode=Two Bit Locations  nbits=CoeffBitWidth * (TotalTaps - 1)  bit1=0  base1=MSB of Input  bit0=CoeffBitWidth  base0=LSB of Input  boolean_output=off  explicit_period=off  period=1  dbl_ovrd=off
  delay : Subsystem  BlockChoice=delay_bram
      link override delay_bram: DelayLen=2^(PFBSize-n_inputs)  bram_latency=bram_latency
      link override delay_bram/Constant2: equ=P=C
      settings: AttributesFormatString=%<BlockChoice>  TemplateBlock=casper_library/Delays/delay  MemberBlocks=delay_bram,delay_slr
  pfb_coeff_gen : Subsystem  AncestorBlock=casper_library/PFBs/pfb_coeff_gen  mask(pfb_coeff_gen){PFBSize=5, CoeffBitWidth=8, TotalTaps=2, CoeffDistMem=1, CoeffRound=0, WindowType=hamming, bram_latency=2, n_inputs=2, nput=2, fwidth=1}
      mask prompts: PFBSize "Size of PFB: (2^? pnts)"; CoeffBitWidth "Bitwidth of Coefficients:"; TotalTaps "Total Number of Taps:"; CoeffDistMem "Implement Coeff Gen in Distributed Memory"; CoeffRound "Round-off Coefficients"; WindowType "Windowing Function:"; bram_latency "BRAM Latency"; n_inputs "Number of Simultaneous Inputs: (2^?)"; nput "This is input number:"; fwidth "Bin Width (normal=1)"
      mask init: same as pasp_16i16c128s/pasp/pfb_fir_real/pol1_in1_first_tap/pfb_coeff_gen
      settings: AttributesFormatString=PFBSize=5, n_inputs=2, taps=2
  sync_delay : casper_library/Delays/sync_delay  DelayLen=2^(PFBSize-n_inputs)
      link override Constant: equ=P=C
      link override Constant1: equ=P=C
      link override Constant2: equ=P=C
      link override Constant3: equ=P=C
  dout : Outport
  sync_out : Outport  Port=2
  coeff_out : Outport  Port=3
  taps_out : Outport  Port=4
  wires:
  Reinterpret2/1 -> Mult/1
  Reinterpret1/1 -> taps_out/1
  Reinterpret/1 -> Mult/2
  Slice/1 -> Reinterpret/1
  Slice1/1 -> coeff_out/1
  sync_delay/1 -> sync_out/1
  delay/1(Out1) -> dout/1
  pfb_coeff_gen/1(dout) -> delay/1(In1), Reinterpret2/1
  pfb_coeff_gen/2(sync_out) -> sync_delay/1
  pfb_coeff_gen/3(coeff) -> Slice/1, Slice1/1
  Mult/1 -> Reinterpret1/1
  din/1 -> pfb_coeff_gen/1(din)
  sync/1 -> pfb_coeff_gen/2(sync)

== system pasp_16i16c128s/pasp/pfb_fir_real1/pol1_in3_last_tap ==
  din : Inport  Port=1  LatchInput=off
  sync : Inport  Port=2  LatchInput=off
  coeff : Inport  Port=3  LatchInput=off
  taps : Inport  Port=4  LatchInput=off
  Concat : xbsIndex_r3/Concat  num_inputs=2  explicit_period=off  period=1  dbl_ovrd=off
  Delay : xbsIndex_r3/Delay  latency=mult_latency  reg_retiming=off  explicit_period=off  period=1  en=off  accept_only_valid=off  init_zero=on  dbl_ovrd=off  show_param=off
      settings: xl_area=[0, 0, 0, 0, 0, 0, 0]
  Mult : xbsIndex_r3/Mult  precision=Full  arith_type="Signed  (2's comp)"  n_bits=8  bin_pt=2  quantization=Truncate  overflow=Wrap  latency=mult_latency  explicit_period=off  period=1  en=off  dbl_ovrd=off  show_param=on  mult_type=Parallel  oversample=2  use_embedded=on  pipeline=on  use_rpm=on  placement_style=Rectangular Shape  gen_core=off
      settings: xl_area=[0, 0, 0, 0, 0, 0, 0]
  Reinterpret : xbsIndex_r3/Reinterpret  force_arith_type=on  arith_type="Signed  (2's comp)"  force_bin_pt=on  bin_pt=CoeffBitWidth - 1  force_valid=on
  Reinterpret1 : xbsIndex_r3/Reinterpret  force_arith_type=on  arith_type="Signed  (2's comp)"  force_bin_pt=on  bin_pt=BitWidthIn - 1  force_valid=on
  Reinterpret2 : xbsIndex_r3/Reinterpret  force_arith_type=on  arith_type=Unsigned  force_bin_pt=on  bin_pt=0  force_valid=on
  pfb_real_add_tree : Subsystem  mask(pfb_real_add_tree){TotalTaps=2, BitWidthIn=8, BitWidthOut=18, CoeffBitWidth=8, add_latency=1, quantization=Truncate}
      mask prompts: TotalTaps "Total Number of Taps:"; BitWidthIn "Input Bitwidth:"; BitWidthOut "Output Bitwidth:"; CoeffBitWidth "Coeff Bitwidth:"; add_latency "Add Latency"; quantization "Quantization Behavior"
      mask init: same as pasp_16i16c128s/pasp/pfb_fir_real/pol1_in1_last_tap/pfb_real_add_tree
      settings: AttributesFormatString=taps=2, add_latency=1
  dout : Outport
  sync_out : Outport  Port=2
  wires:
  Delay/1 -> pfb_real_add_tree/2(sync)
  pfb_real_add_tree/2(sync_out) -> sync_out/1
  din/1 -> Reinterpret1/1
  sync/1 -> Delay/1
  taps/1 -> Concat/2
  Concat/1 -> pfb_real_add_tree/1(din)
  coeff/1 -> Reinterpret/1
  Reinterpret/1 -> Mult/2
  Mult/1 -> Reinterpret2/1
  Reinterpret1/1 -> Mult/1
  Reinterpret2/1 -> Concat/1
  pfb_real_add_tree/1(dout) -> dout/1

== system pasp_16i16c128s/pasp/pfb_fir_real1/pol1_in4_first_tap ==
  din : Inport  Port=1  LatchInput=off
  sync : Inport  Port=2  LatchInput=off
  Mult : xbsIndex_r3/Mult  precision=Full  arith_type="Signed  (2's comp)"  n_bits=8  bin_pt=2  quantization=Truncate  overflow=Wrap  latency=mult_latency  explicit_period=off  period=1  en=off  dbl_ovrd=off  show_param=on  mult_type=Parallel  oversample=2  use_embedded=on  pipeline=on  use_rpm=on  placement_style=Rectangular Shape  gen_core=off
      settings: xl_area=[0, 0, 0, 0, 0, 0, 0]
  Reinterpret : xbsIndex_r3/Reinterpret  force_arith_type=on  arith_type="Signed  (2's comp)"  force_bin_pt=on  bin_pt=CoeffBitWidth - 1  force_valid=on
  Reinterpret1 : xbsIndex_r3/Reinterpret  force_arith_type=on  arith_type=Unsigned  force_bin_pt=on  bin_pt=0  force_valid=on
  Reinterpret2 : xbsIndex_r3/Reinterpret  force_arith_type=on  arith_type="Signed  (2's comp)"  force_bin_pt=on  bin_pt=BitWidthIn - 1  force_valid=on
  Slice : xbsIndex_r3/Slice  mode=Lower Bit Location + Width  nbits=CoeffBitWidth  bit1=0  base1=MSB of Input  bit0=0  base0=LSB of Input  boolean_output=off  explicit_period=off  period=1  dbl_ovrd=off
  Slice1 : xbsIndex_r3/Slice  mode=Two Bit Locations  nbits=CoeffBitWidth * (TotalTaps - 1)  bit1=0  base1=MSB of Input  bit0=CoeffBitWidth  base0=LSB of Input  boolean_output=off  explicit_period=off  period=1  dbl_ovrd=off
  delay : Subsystem  BlockChoice=delay_bram
      link override delay_bram: DelayLen=2^(PFBSize-n_inputs)  bram_latency=bram_latency
      link override delay_bram/Constant2: equ=P=C
      settings: AttributesFormatString=%<BlockChoice>  TemplateBlock=casper_library/Delays/delay  MemberBlocks=delay_bram,delay_slr
  pfb_coeff_gen : Subsystem  AncestorBlock=casper_library/PFBs/pfb_coeff_gen  mask(pfb_coeff_gen){PFBSize=5, CoeffBitWidth=8, TotalTaps=2, CoeffDistMem=1, CoeffRound=0, WindowType=hamming, bram_latency=2, n_inputs=2, nput=3, fwidth=1}
      mask prompts: PFBSize "Size of PFB: (2^? pnts)"; CoeffBitWidth "Bitwidth of Coefficients:"; TotalTaps "Total Number of Taps:"; CoeffDistMem "Implement Coeff Gen in Distributed Memory"; CoeffRound "Round-off Coefficients"; WindowType "Windowing Function:"; bram_latency "BRAM Latency"; n_inputs "Number of Simultaneous Inputs: (2^?)"; nput "This is input number:"; fwidth "Bin Width (normal=1)"
      mask init: same as pasp_16i16c128s/pasp/pfb_fir_real/pol1_in1_first_tap/pfb_coeff_gen
      settings: AttributesFormatString=PFBSize=5, n_inputs=2, taps=2
  sync_delay : casper_library/Delays/sync_delay  DelayLen=2^(PFBSize-n_inputs)
      link override Constant: equ=P=C
      link override Constant1: equ=P=C
      link override Constant2: equ=P=C
      link override Constant3: equ=P=C
  dout : Outport
  sync_out : Outport  Port=2
  coeff_out : Outport  Port=3
  taps_out : Outport  Port=4
  wires:
  Reinterpret2/1 -> Mult/1
  Reinterpret1/1 -> taps_out/1
  Reinterpret/1 -> Mult/2
  Slice/1 -> Reinterpret/1
  Slice1/1 -> coeff_out/1
  sync_delay/1 -> sync_out/1
  delay/1(Out1) -> dout/1
  pfb_coeff_gen/1(dout) -> delay/1(In1), Reinterpret2/1
  pfb_coeff_gen/2(sync_out) -> sync_delay/1
  pfb_coeff_gen/3(coeff) -> Slice/1, Slice1/1
  Mult/1 -> Reinterpret1/1
  din/1 -> pfb_coeff_gen/1(din)
  sync/1 -> pfb_coeff_gen/2(sync)

== system pasp_16i16c128s/pasp/pfb_fir_real1/pol1_in4_last_tap ==
  din : Inport  Port=1  LatchInput=off
  sync : Inport  Port=2  LatchInput=off
  coeff : Inport  Port=3  LatchInput=off
  taps : Inport  Port=4  LatchInput=off
  Concat : xbsIndex_r3/Concat  num_inputs=2  explicit_period=off  period=1  dbl_ovrd=off
  Delay : xbsIndex_r3/Delay  latency=mult_latency  reg_retiming=off  explicit_period=off  period=1  en=off  accept_only_valid=off  init_zero=on  dbl_ovrd=off  show_param=off
      settings: xl_area=[0, 0, 0, 0, 0, 0, 0]
  Mult : xbsIndex_r3/Mult  precision=Full  arith_type="Signed  (2's comp)"  n_bits=8  bin_pt=2  quantization=Truncate  overflow=Wrap  latency=mult_latency  explicit_period=off  period=1  en=off  dbl_ovrd=off  show_param=on  mult_type=Parallel  oversample=2  use_embedded=on  pipeline=on  use_rpm=on  placement_style=Rectangular Shape  gen_core=off
      settings: xl_area=[0, 0, 0, 0, 0, 0, 0]
  Reinterpret : xbsIndex_r3/Reinterpret  force_arith_type=on  arith_type="Signed  (2's comp)"  force_bin_pt=on  bin_pt=CoeffBitWidth - 1  force_valid=on
  Reinterpret1 : xbsIndex_r3/Reinterpret  force_arith_type=on  arith_type="Signed  (2's comp)"  force_bin_pt=on  bin_pt=BitWidthIn - 1  force_valid=on
  Reinterpret2 : xbsIndex_r3/Reinterpret  force_arith_type=on  arith_type=Unsigned  force_bin_pt=on  bin_pt=0  force_valid=on
  pfb_real_add_tree : Subsystem  mask(pfb_real_add_tree){TotalTaps=2, BitWidthIn=8, BitWidthOut=18, CoeffBitWidth=8, add_latency=1, quantization=Truncate}
      mask prompts: TotalTaps "Total Number of Taps:"; BitWidthIn "Input Bitwidth:"; BitWidthOut "Output Bitwidth:"; CoeffBitWidth "Coeff Bitwidth:"; add_latency "Add Latency"; quantization "Quantization Behavior"
      mask init: same as pasp_16i16c128s/pasp/pfb_fir_real/pol1_in1_last_tap/pfb_real_add_tree
      settings: AttributesFormatString=taps=2, add_latency=1
  dout : Outport
  sync_out : Outport  Port=2
  wires:
  Delay/1 -> pfb_real_add_tree/2(sync)
  pfb_real_add_tree/2(sync_out) -> sync_out/1
  din/1 -> Reinterpret1/1
  sync/1 -> Delay/1
  taps/1 -> Concat/2
  Concat/1 -> pfb_real_add_tree/1(din)
  coeff/1 -> Reinterpret/1
  Reinterpret/1 -> Mult/2
  Mult/1 -> Reinterpret2/1
  Reinterpret1/1 -> Mult/1
  Reinterpret2/1 -> Concat/1
  pfb_real_add_tree/1(dout) -> dout/1
